simulink library "ddm"  (R2021b)
settings: Solver=VariableStepAuto  StartTime=0.0  StopTime=10.0  RelTol=1e-3
undefined symbols (not defined in the file): ADDM_FrTMTqDev_X_Nm, ADDM_RrTMTqDev_X_Nm, ENUM_ADASACCSTA_ERROR, ENUM_ADASACCSTA_OFF, ENUM_ADASACCSTA_STANDBY, ENUM_ALLOWMOV_ALLOWREADY, ENUM_APS, ENUM_BRKSTA_ERROR, ENUM_BRKSTA_OFF, ENUM_BRKSTA_ON, ENUM_BRKSW_INVALID, ENUM_BRKSW_OFF, ENUM_BRKSW_ON, ENUM_CHGPREACTERRSTA_OBCPRE, ENUM_DCDCFAULTSTA_ANYFAULTLV1, ENUM_DCDCFAULTSTA_ANYFAULTLV2, ENUM_DRIVETRAIN_AWD, ENUM_DRIVETRAIN_FWD, ENUM_DRIVETRAIN_RWD, ENUM_EDUDRTSTA_NORMAL, ENUM_EPBERROR_FAILED, ENUM_EPBSTA_APPLIED, ENUM_EPBSTA_RELEASED, ENUM_ESCAPSSta_APSUNAVAILABLE, ENUM_GEARACTUALPOSN_INVALID, ENUM_GEARACTUALPOSN_P, ENUM_HVBATTREADYPRE_READY, ENUM_HWRESETSTA_HWRESETING, ENUM_MCUWARN_LV0, ENUM_MCUWARN_LV1, ENUM_MCUWARN_LV2, ENUM_MCUWARN_LV3, ENUM_MCUWARN_NOERROR, ENUM_OBCFAULTSTA_ANYFAULT, ENUM_PAS_R2F2, ENUM_PDFAULT_BATTPDFAIL, ENUM_PDFAULT_DCDCDISABLE, ENUM_PDFAULT_MCUDISABLE, ENUM_PDFAULT_MCUDISCHRG, ENUM_POWERSTA_OFF, ENUM_POWERSTA_ON, ENUM_POWERSTA_READY, ENUM_POWERSTA_STANDBY, ENUM_PRESSINDI_LOW, ENUM_PUFAULT_BATTUPFAIL, ENUM_PUFAULT_DCDCENABLEFAIL, ENUM_PUFAULT_PRECHRGCHKFAIL, ENUM_PUFAULT_SAFETYCHKFAIL, ENUM_PWRSTASW_OFF, ENUM_PWRSTASW_OFFA, ENUM_PWRSTASW_OFFCHVCHRG, ENUM_PWRSTASW_OFFCLVCHRG, ENUM_PWRSTASW_ON, ENUM_PWRSTASW_ONHVCHRG, ENUM_PWRSTASW_READY, ENUM_PWRSTASW_STANDBY, ENUM_RAPSErrWarnSta_NORMAL, ENUM_RAPSErrWarnSta_RAPSERRLV1, ENUM_SHIFTCOMMAND_P, ENUM_SHIFTERERRSTA_PBUTTONFAILURE ... (+471)
libraries: hcu_lib x540, simulink x3
(part 14 of 26)

== system ddm/DDM/DDM/TQD/ESC5_DDM ==
  note: Release Condition After Decision
  note: Diagnostics and Fault Handling
  note: Diagnostics and Fault Handling
  note: Release Condition After Decision
  note: Diagnostics and Fault Handling
  note: Release Condition After Decision
  note: ESC5 CheckSum Error (ESC5CSErr)
  note: ESC5 Rolling Count Error (ESC5RCErr)
  note: ESC5 Lost Comm (ESC5NoCom)
  task_time_s : Inport
  VPMM_SysPwrSta_enum : Inport  Port=2
  No_CAN1_BUS_OFF : Inport  Port=3
  VDDM_ESC5NoCom_flg : Inport  Port=4
  VDDM_ESC5RCErr_flg : Inport  Port=5
  VDDM_ESC5CSErr_flg : Inport  Port=6
  DTC_clear_request : Inport  Port=7
  Constant{1,3..5,11,15,18,22,48} (9 alike) : Constant  Value=ENUM_PWRSTASW_OFF
  Constant10 : Constant  Value=ENUM_PWRSTASW_STANDBY
  Constant101 : Constant  Value=KDDM_TQDDiagnosisOffSW_flg
  Constant102 : Constant  Value=ZERO_INT
  Constant12 : Constant  Value=FALSE
  Constant13 : Constant  Value=KDDM_ESC5RCErrDTC_cnt
  Constant14 : Constant  Value=KDDM_ESC5RCErrPassTO_s
  Constant17 : Constant  Value=KDDM_ESC5CSErrDTC_cnt
  Constant2 : Constant  Value=KDDM_ESC5NoComDTC_cnt
  Constant20 : Constant  Value=KDDM_TQDDiagnosisOffSW_flg
  Constant21 : Constant  Value=ENUM_PWRSTASW_STANDBY
  Constant25 : Constant  Value=KDDM_ESC5RCErrDetTO_s
  Constant27 : Constant  Value=FALSE
  Constant28 : Constant  Value=KDDM_ESC5NoComDTC_cnt
  Constant29 : Constant  Value=KDDM_ESC5NoComPassTO_s
  Constant30 : Constant  Value=KDDM_ESC5NoComDetTO_s
  Constant35 : Constant  Value=KDDM_ESC5RCErrPassTO_s
  Constant41 : Constant  Value=FALSE
  Constant42 : Constant  Value=KDDM_ESC5CSErrDTC_cnt
  Constant43 : Constant  Value=KDDM_ESC5CSErrPassTO_s
  Constant44 : Constant  Value=KDDM_ESC5CSErrDetTO_s
  Constant45 : Constant  Value=ZERO_INT
  Constant51 : Constant  Value=KDDM_ESC5CSErrPassTO_s
  Constant55 : Constant  Value=KDDM_ESC5NoComPassTO_s
  Constant6 : Constant  Value=KDDM_ESC5RCErrDTC_cnt
  Constant7 : Constant  Value=KDDM_TQDDiagnosisOffSW_flg
  Constant8 : Constant  Value=ZERO_INT
  Constant9 : Constant  Value=ENUM_PWRSTASW_STANDBY
  DTC_Couter1 : hcu_lib/Basic_Blocks/DTC_Couter
  DTC_Couter2 : hcu_lib/Basic_Blocks/DTC_Couter
  DTC_Couter7 : hcu_lib/Basic_Blocks/DTC_Couter
  DTC_Info1 : hcu_lib/Basic_Blocks/DTC_Info
  DTC_Info2 : hcu_lib/Basic_Blocks/DTC_Info
  DTC_Info3 : hcu_lib/Basic_Blocks/DTC_Info
  Delay1 : Delay  DelayLength=1
  Delay2 : Delay  DelayLength=1
  Delay3 : Delay  DelayLength=1
  Equal{1,7,19,23,49..50} (6 alike) : RelationalOperator  Operator===  OutDataTypeStr=boolean  RndMeth=Simplest
  Equal15 : RelationalOperator  OutDataTypeStr=boolean  RndMeth=Simplest
  Equal{2..6,8} (6 alike) : RelationalOperator  Operator=~=  OutDataTypeStr=boolean  RndMeth=Simplest
  Equal20 : RelationalOperator  OutDataTypeStr=boolean  RndMeth=Simplest
  Equal21 : RelationalOperator  OutDataTypeStr=boolean  RndMeth=Simplest
  Logical Operator : Logic  Operator=OR  Inputs=3  AllPortsSameDT=off  OutDataTypeStr=boolean
  Logical Operator1 : Logic  Operator=OR  Inputs=4  AllPortsSameDT=off  OutDataTypeStr=boolean
  Logical Operator{11..13,19,26,30,37,41,45,53} (10 alike) : Logic  Operator=NOT  AllPortsSameDT=off  OutDataTypeStr=boolean
  Logical Operator{2,5..6,8,54..55} (6 alike) : Logic  AllPortsSameDT=off  OutDataTypeStr=boolean
  Logical Operator{28,32,43,46} (4 alike) : Logic  Inputs=4  AllPortsSameDT=off  OutDataTypeStr=boolean
  Logical Operator3 : Logic  Operator=OR  Inputs=4  AllPortsSameDT=off  OutDataTypeStr=boolean
  Logical Operator4 : Logic  Inputs=3  AllPortsSameDT=off  OutDataTypeStr=boolean
  Logical Operator49 : Logic  Operator=OR  Inputs=4  AllPortsSameDT=off  OutDataTypeStr=boolean
  Logical Operator50 : Logic  Inputs=3  AllPortsSameDT=off  OutDataTypeStr=boolean
  NOT1 : Logic  Operator=NOT  AllPortsSameDT=off  OutDataTypeStr=boolean
  NOT2 : Logic  Operator=NOT  AllPortsSameDT=off  OutDataTypeStr=boolean
  NOT3 : Logic  Operator=NOT  AllPortsSameDT=off  OutDataTypeStr=boolean
  Relational Operator1 : RelationalOperator  Operator=>  OutDataTypeStr=boolean  RndMeth=Simplest
  Relational Operator2 : RelationalOperator  Operator=>  OutDataTypeStr=boolean  RndMeth=Simplest
  Relational Operator3 : RelationalOperator  Operator=>  OutDataTypeStr=boolean  RndMeth=Simplest
  Switch1 : Switch  Criteria=u2 ~= 0
  Switch2 : Switch  Criteria=u2 ~= 0
  Switch3 : Switch  Criteria=u2 ~= 0
  Terminator : Terminator
  Terminator1 : Terminator
  Terminator2 : Terminator
  Test Detection Criteria2 : hcu_lib/Basic_Blocks/Test Detection Criteria
  Test Detection Criteria3 : hcu_lib/Basic_Blocks/Test Detection Criteria
  Test Detection Criteria4 : hcu_lib/Basic_Blocks/Test Detection Criteria
  Timer1 : hcu_lib/Basic_Blocks/Timer
  Timer3 : hcu_lib/Basic_Blocks/Timer
  Timer4 : hcu_lib/Basic_Blocks/Timer
  Unit Delay1 : UnitDelay  SampleTime=-1  HasFrameUpgradeWarning=on
  Unit Delay6 : UnitDelay  SampleTime=-1  HasFrameUpgradeWarning=on
  Unit Delay7 : UnitDelay  SampleTime=-1  HasFrameUpgradeWarning=on
  VDDM_ESC5NoComDTC_raw32 : Outport
  VDDM_ESC5RCErrDTC_raw32 : Outport  Port=2
  VDDM_ESC5CSErrDTC_raw32 : Outport  Port=3
  VDDM_ESC5NoComCFS_flg : Outport  Port=4
  VDDM_ESC5RCErrCFS_flg : Outport  Port=5
  VDDM_ESC5CSErrCFS_flg : Outport  Port=6
  VDDM_ESC5Err_flg : Outport  Port=7
  wires:
  [VPMM_SysPwrSta_enum] -> Equal8/1
  Constant15/1 -> Equal8/2
  [VPMM_SysPwrSta_enum] -> Equal5/1
  Constant11/1 -> Equal5/2
  Equal7/1 -> Logical Operator2/1
  [VDDM_ESC5CSErrCFS_flg] -> Delay2/1
  Constant18/1 -> Equal7/2
  DTC_Couter2/2 -> Relational Operator1/1  "VDDM_ESC5CSErrDTC_cnt"
  [VDDM_ESC5CSErrCFSRls_flg] -> DTC_Couter2/2
  [DTC_clear_request] -> Logical Operator1/2
  Equal1/1 -> Logical Operator2/2
  Delay2/1 -> NOT2/1
  Logical Operator6/1 -> Logical Operator1/3
  Constant8/1 -> Relational Operator1/2
  Constant7/1 -> Logical Operator1/4
  Unit Delay1/1 -> Equal7/1
  Relational Operator1/1 -> Terminator2/1  "VDDM_ESC5CSErrDFS_flg"
  [VDDM_ESC5CSErrPass_flg] -> Logical Operator6/1
  DTC_Couter2/1 -> [VDDM_ESC5CSErrCFS_flg]  "VDDM_ESC5CSErrCFS_flg"
  [VPMM_SysPwrSta_enum] -> Unit Delay1/1
  Logical Operator2/1 -> Logical Operator1/1
  Constant10/1 -> Equal1/2
  NOT2/1 -> Logical Operator6/2
  [VPMM_SysPwrSta_enum] -> Equal1/1
  Constant17/1 -> DTC_Couter2/3
  Logical Operator1/1 -> [VDDM_ESC5CSErrCFSRls_flg]  "VDDM_ESC5CSErrCFSRls_flg"
  [VDDM_ESC5CSErrDet_flg] -> DTC_Couter2/1
  Equal49/1 -> Logical Operator5/2
  [VPMM_SysPwrSta_enum] -> Equal49/1
  NOT3/1 -> Logical Operator8/2
  DTC_Couter7/1 -> [VDDM_ESC5RCErrCFS_flg]  "VDDM_ESC5RCErrCFS_flg"
  Constant9/1 -> Equal49/2
  [VPMM_SysPwrSta_enum] -> Unit Delay7/1
  Equal50/1 -> Logical Operator5/1
  Relational Operator3/1 -> Terminator1/1  "VDDM_ESC5RCErrDFS_flg"
  [VDDM_ESC5RCErrPass_flg] -> Logical Operator8/1
  Logical Operator5/1 -> Logical Operator3/1
  [VDDM_ESC5RCErrCFS_flg] -> Delay3/1
  Logical Operator8/1 -> Logical Operator3/3
  Constant101/1 -> Logical Operator3/4
  [DTC_clear_request] -> Logical Operator3/2
  Constant102/1 -> Relational Operator3/2
  Constant6/1 -> DTC_Couter7/3
  [VDDM_ESC5RCErrDet_flg] -> DTC_Couter7/1
  Logical Operator3/1 -> [VDDM_ESC5RCErrCFSRls_flg]  "VDDM_ESC5RCErrCFSRls_flg"
  DTC_Couter7/2 -> Relational Operator3/1  "VDDM_ESC5RCErrDTC_cnt"
  Delay3/1 -> NOT3/1
  [VDDM_ESC5RCErrCFSRls_flg] -> DTC_Couter7/2
  Constant22/1 -> Equal50/2
  Unit Delay7/1 -> Equal50/1
  Constant5/1 -> Equal6/2
  [VPMM_SysPwrSta_enum] -> Equal6/1
  Constant4/1 -> Equal4/2
  [VPMM_SysPwrSta_enum] -> Equal4/1
  [VPMM_SysPwrSta_enum] -> Equal3/1
  Constant1/1 -> Equal3/2
  [VPMM_SysPwrSta_enum] -> Equal2/1
  Constant3/1 -> Equal2/2
  Equal19/1 -> Logical Operator55/2
  [VDDM_ESC5NoComPass_flg] -> Logical Operator54/1
  Constant2/1 -> DTC_Couter1/3
  [VDDM_ESC5NoComCFS_flg] -> Delay1/1
  DTC_Couter1/2 -> Relational Operator2/1  "VDDM_ESC5NoComDTC_cnt"
  DTC_Couter1/1 -> [VDDM_ESC5NoComCFS_flg]  "VDDM_ESC5NoComCFS_flg"
  Constant21/1 -> Equal19/2
  Equal23/1 -> Logical Operator55/1
  [VPMM_SysPwrSta_enum] -> Equal19/1
  [VDDM_ESC5NoComCFSRls_flg] -> DTC_Couter1/2
  [VDDM_ESC5NoComDet_flg] -> DTC_Couter1/1
  Constant48/1 -> Equal23/2
  Unit Delay6/1 -> Equal23/1
  Logical Operator49/1 -> [VDDM_ESC5NoComCFSRls_flg]  "VDDM_ESC5NoComCFSRls_flg"
  [DTC_clear_request] -> Logical Operator49/2
  Constant45/1 -> Relational Operator2/2
  Relational Operator2/1 -> Terminator/1  "VDDM_ESC5NoComDFS_flg"
  Logical Operator54/1 -> Logical Operator49/3
  Delay1/1 -> NOT1/1
  NOT1/1 -> Logical Operator54/2
  Constant20/1 -> Logical Operator49/4
  Logical Operator55/1 -> Logical Operator49/1
  [VPMM_SysPwrSta_enum] -> Unit Delay6/1
  [VDDM_ESC5CSErrCFS_flg] -> VDDM_ESC5CSErrCFS_flg/1
  [VDDM_ESC5RCErrCFS_flg] -> VDDM_ESC5RCErrCFS_flg/1
  [VDDM_ESC5NoComCFS_flg] -> VDDM_ESC5NoComCFS_flg/1
  [VDDM_ESC5NoComCFS_flg] -> Logical Operator13/1
  Logical Operator13/1 -> Logical Operator43/4
  [VDDM_ESC5NoComCFS_flg] -> Logical Operator11/1
  Logical Operator11/1 -> Logical Operator28/4
  VDDM_ESC5CSErr_flg/1 -> [VDDM_ESC5CSErr_flg]
  VDDM_ESC5RCErr_flg/1 -> [VDDM_ESC5RCErr_flg]
  [VDDM_ESC5NoCom_flg] -> Logical Operator4/3
  Test Detection Criteria2/1 -> [VDDM_ESC5NoComDet_flg]  "VDDM_ESC5NoComDet_flg"
  Logical Operator37/1 -> Timer4/2
  Test Detection Criteria3/1 -> [VDDM_ESC5RCErrDet_flg]  "VDDM_ESC5RCErrDet_flg"
  [No_CAN1_BUS_OFF] -> Logical Operator32/2
  [No_CAN1_BUS_OFF] -> Logical Operator50/2
  [VDDM_ESC5NoCom_flg] -> Logical Operator53/1
  [VDDM_ESC5NoComPass_flg] -> DTC_Info1/2
  VDDM_ESC5NoCom_flg/1 -> [VDDM_ESC5NoCom_flg]
  Switch3/1 -> Test Detection Criteria2/1
  Timer4/1 -> Equal15/1
  Logical Operator41/1 -> Logical Operator32/4
  [VDDM_ESC5RCErr_flg] -> Logical Operator30/1
  Logical Operator19/1 -> Timer3/2
  Equal21/1 -> [VDDM_ESC5RCErrPass_flg]  "VDDM_ESC5RCErrPass_flg"
  Logical Operator43/1 -> Logical Operator37/1, Timer4/1
  Logical Operator53/1 -> Logical Operator50/3
  Logical Operator46/1 -> Switch1/3
  Constant44/1 -> Test Detection Criteria4/4
  [VDDM_ESC5CSErrCFS_flg] -> DTC_Info3/3
  Logical Operator26/1 -> Logical Operator46/4
  [VDDM_ESC5RCErrCFSRls_flg] -> Switch1/2
  [task_time_s] -> Timer4/3
  Constant12/1 -> Switch1/1
  Logical Operator12/1 -> Timer1/2
  [No_CAN1_BUS_OFF] -> Logical Operator4/2
  Logical Operator4/1 -> Switch3/3
  [task_time_s] -> Test Detection Criteria3/2
  [VDDM_ESC5RCErrDet_flg] -> DTC_Info2/1
  [task_time_s] -> Test Detection Criteria4/2
  Logical Operator28/1 -> Logical Operator12/1, Timer1/1
  Equal2/1 -> Logical Operator4/1
  DTC_Info1/1 -> VDDM_ESC5NoComDTC_raw32/1  "VDDM_ESC5NoComDTC_raw32"
  Constant13/1 -> Test Detection Criteria3/3
  Test Detection Criteria4/1 -> [VDDM_ESC5CSErrDet_flg]  "VDDM_ESC5CSErrDet_flg"
  Switch1/1 -> Test Detection Criteria3/1
  [VDDM_ESC5RCErr_flg] -> Logical Operator46/3
  Equal5/1 -> Logical Operator32/1
  [VDDM_ESC5CSErrDet_flg] -> DTC_Info3/1
  Logical Operator50/1 -> Timer3/1, Logical Operator19/1
  No_CAN1_BUS_OFF/1 -> [No_CAN1_BUS_OFF]
  [VDDM_ESC5NoComCFS_flg] -> Logical Operator26/1
  [DTC_clear_request] -> DTC_Info3/4
  Equal3/1 -> Logical Operator50/1
  [VDDM_ESC5CSErrCFSRls_flg] -> Switch2/2
  Constant42/1 -> Test Detection Criteria4/3
  [VDDM_ESC5NoComCFS_flg] -> Logical Operator41/1
  DTC_clear_request/1 -> [DTC_clear_request]
  [VDDM_ESC5RCErrCFS_flg] -> DTC_Info2/3
  Constant35/1 -> Timer1/4
  Logical Operator30/1 -> Logical Operator28/3
  Timer1/1 -> Equal21/1
  [VDDM_ESC5NoComDet_flg] -> DTC_Info1/1
  Equal6/1 -> Logical Operator28/1
  [No_CAN1_BUS_OFF] -> Logical Operator28/2
  Constant14/1 -> Equal21/2
  Logical Operator32/1 -> Switch2/3
  Equal20/1 -> [VDDM_ESC5NoComPass_flg]  "VDDM_ESC5NoComPass_flg"
  [VDDM_ESC5RCErrPass_flg] -> DTC_Info2/2
  [task_time_s] -> Timer1/3
  [VDDM_ESC5NoComCFSRls_flg] -> Switch3/2
  VPMM_SysPwrSta_enum/1 -> [VPMM_SysPwrSta_enum]
  Equal4/1 -> Logical Operator46/1
  Constant51/1 -> Timer4/4
  Switch2/1 -> Test Detection Criteria4/1
  [VDDM_ESC5CSErrPass_flg] -> DTC_Info3/2
  Equal15/1 -> [VDDM_ESC5CSErrPass_flg]  "VDDM_ESC5CSErrPass_flg"
  Constant43/1 -> Equal15/2
  Constant30/1 -> Test Detection Criteria2/4
  Constant28/1 -> Test Detection Criteria2/3
  [DTC_clear_request] -> DTC_Info2/4
  Constant25/1 -> Test Detection Criteria3/4
  [task_time_s] -> Timer3/3
  DTC_Info3/1 -> VDDM_ESC5CSErrDTC_raw32/1  "VDDM_ESC5CSErrDTC_raw32"
  [task_time_s] -> Test Detection Criteria2/2
  [VDDM_ESC5NoComCFS_flg] -> DTC_Info1/3
  [No_CAN1_BUS_OFF] -> Logical Operator43/2
  [VDDM_ESC5CSErr_flg] -> Logical Operator45/1
  DTC_Info2/1 -> VDDM_ESC5RCErrDTC_raw32/1  "VDDM_ESC5RCErrDTC_raw32"
  Equal8/1 -> Logical Operator43/1
  task_time_s/1 -> [task_time_s]
  Constant27/1 -> Switch3/1
  Constant29/1 -> Equal20/2
  Logical Operator45/1 -> Logical Operator43/3
  Constant41/1 -> Switch2/1
  [No_CAN1_BUS_OFF] -> Logical Operator46/2
  [DTC_clear_request] -> DTC_Info1/4
  Timer3/1 -> Equal20/1
  Constant55/1 -> Timer3/4
  [VDDM_ESC5CSErr_flg] -> Logical Operator32/3
  [VDDM_ESC5RCErrCFS_flg] -> Logical Operator/2
  [VDDM_ESC5NoComCFS_flg] -> Logical Operator/1
  [VDDM_ESC5CSErrCFS_flg] -> Logical Operator/3
  Logical Operator/1 -> VDDM_ESC5Err_flg/1  "VDDM_ESC5Err_flg"

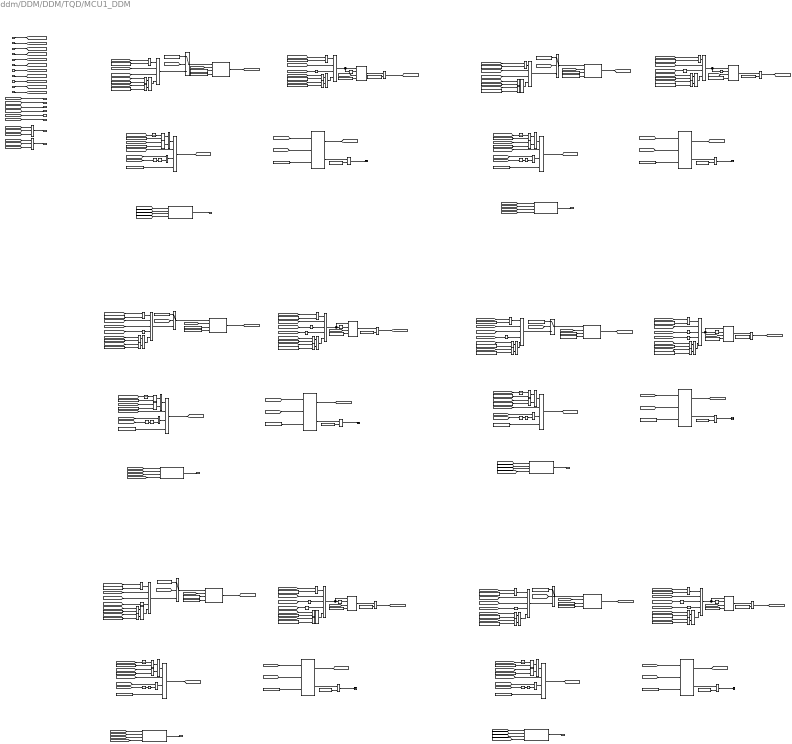
== system ddm/DDM/DDM/TQD/MCU1_DDM ==
  note: Diagnostics and Fault Handling
  note: Release Condition After Decision
  note: Diagnostics and Fault Handling
  note: Release Condition After Decision
  note: Diagnostics and Fault Handling
  note: Release Condition After Decision
  note: Release Condition After Decision
  note: Diagnostics and Fault Handling
  note: Release Condition After Decision
  note: Diagnostics and Fault Handling
  note: Release Condition After Decision
  note: Diagnostics and Fault Handling
  note: MCU_F1 Lost Comm (MCUF1NoCom)
  note: MCU_R1 Lost Comm (MCUR1NoCom)
  note: MCU_R1 Rolling Count Error (MCUR1RCErr)
  note: MCU_F1 Rolling Count Error (MCUF1RCErr)
  note: MCU_R1 Checksum Error (MCUR1CSErr)
  note: MCU_F1 Checksum Error (MCUF1CSErr)
  task_time_s : Inport
  VPMM_SysPwrSta_enum : Inport  Port=2
  No_CAN3_BUS_OFF : Inport  Port=3
  VDDM_MCUF1NoCom_flg : Inport  Port=4
  VDDM_MCUR1NoCom_flg : Inport  Port=5
  VDDM_MCUF1RCErr_flg : Inport  Port=6
  VDDM_MCUF1CSErr_flg : Inport  Port=7
  VDDM_MCUR1RCErr_flg : Inport  Port=8
  VDDM_MCUR1CSErr_flg : Inport  Port=9
  DTC_clear_request : Inport  Port=10
  VPMM_DrivetrainSelect_enum : Inport  Port=11
  Constant{1..2,6..7,9,13,26,40,43,46,53,59..60,62,72,75,79,86} (18 alike) : Constant  Value=ENUM_PWRSTASW_OFF
  Constant{3,10,35,41,52,57} (6 alike) : Constant  Value=ENUM_PWRSTASW_STANDBY
  Constant{20,24,28,44,67,88,90,92,94,96,98,100} (12 alike) : Constant  Value=ENUM_DRIVETRAIN_AWD
  Constant{4,11,29,45,55,101} (6 alike) : Constant  Value=KDDM_TQDDiagnosisOffSW_flg
  Constant{5,12,30,49,56,102} (6 alike) : Constant  Value=ZERO_INT
  Constant14 : Constant  Value=KDDM_MCUF1NoComDTC_cnt
  Constant{15,27,66,93,95,97} (6 alike) : Constant  Value=ENUM_DRIVETRAIN_RWD
  Constant16 : Constant  Value=KDDM_MCUR1NoComDTC_cnt
  Constant17 : Constant  Value=KDDM_MCUR1NoComPassTO_s
  Constant18 : Constant  Value=KDDM_MCUR1NoComPassTO_s
  Constant19 : Constant  Value=KDDM_MCUR1NoComDetTO_s
  Constant{21,42,87,89,91,99} (6 alike) : Constant  Value=ENUM_DRIVETRAIN_FWD
  Constant{22..23,38..39,73..74} (6 alike) : Constant  Value=FALSE
  Constant25 : Constant  Value=KDDM_MCUF1RCErrDTC_cnt
  Constant31 : Constant  Value=KDDM_MCUR1RCErrDTC_cnt
  Constant32 : Constant  Value=KDDM_MCUR1RCErrPassTO_s
  Constant33 : Constant  Value=KDDM_MCUR1RCErrPassTO_s
  Constant34 : Constant  Value=KDDM_MCUR1RCErrDetTO_s
  Constant36 : Constant  Value=KDDM_MCUR1RCErrDTC_cnt
  Constant37 : Constant  Value=KDDM_MCUF1CSErrPassTO_s
  Constant47 : Constant  Value=KDDM_MCUF1RCErrDTC_cnt
  Constant48 : Constant  Value=KDDM_MCUF1RCErrPassTO_s
  Constant50 : Constant  Value=KDDM_MCUF1RCErrPassTO_s
  Constant51 : Constant  Value=KDDM_MCUF1RCErrDetTO_s
  Constant54 : Constant  Value=KDDM_MCUF1RCErrDTC_cnt
  Constant58 : Constant  Value=KDDM_MCUR1RCErrDTC_cnt
  Constant61 : Constant  Value=KDDM_MCUR1CSErrDTC_cnt
  Constant63 : Constant  Value=KDDM_MCUR1CSErrPassTO_s
  Constant64 : Constant  Value=KDDM_MCUR1CSErrPassTO_s
  Constant65 : Constant  Value=KDDM_MCUR1CSErrDetTO_s
  Constant68 : Constant  Value=KDDM_MCUF1NoComDTC_cnt
  Constant69 : Constant  Value=KDDM_MCUF1NoComPassTO_s
  Constant70 : Constant  Value=KDDM_MCUF1NoComPassTO_s
  Constant71 : Constant  Value=KDDM_MCUF1NoComDetTO_s
  Constant8 : Constant  Value=KDDM_MCUR1NoComDTC_cnt
  Constant80 : Constant  Value=KDDM_MCUF1CSErrDTC_cnt
  Constant83 : Constant  Value=KDDM_MCUF1CSErrPassTO_s
  Constant84 : Constant  Value=KDDM_MCUF1CSErrDetTO_s
  DTC_Couter{1..5,7} (6 alike) : hcu_lib/Basic_Blocks/DTC_Couter
  DTC_Info{,1..5} (6 alike) : hcu_lib/Basic_Blocks/DTC_Info
  Delay{1..6} (6 alike) : Delay  DelayLength=1
  Equal{,1..4,7..8,12,14..15,19..20,23,26..27,33..43,45,47..55} (36 alike) : RelationalOperator  Operator===  OutDataTypeStr=boolean  RndMeth=Simplest
  Equal{5,9..11,16,18,21..22,24,29,44,46} (12 alike) : RelationalOperator  Operator=~=  OutDataTypeStr=boolean  RndMeth=Simplest
  Equal{6,13,17,25,28,30} (6 alike) : RelationalOperator  OutDataTypeStr=boolean  RndMeth=Simplest
  Logical Operator : Logic  Operator=OR  Inputs=3  AllPortsSameDT=off  OutDataTypeStr=boolean
  Logical Operator{1,3,16,21,33,36} (6 alike) : Logic  Operator=OR  Inputs=4  AllPortsSameDT=off  OutDataTypeStr=boolean
  Logical Operator{6,10,13,15,19..20,24..26,29,32,37,41..42,61,70,81..84} (20 alike) : Logic  Operator=NOT  AllPortsSameDT=off  OutDataTypeStr=boolean
  Logical Operator{4,8..9,11,17..18,22,28,34..35,38..39} (12 alike) : Logic  AllPortsSameDT=off  OutDataTypeStr=boolean
  Logical Operator{7,12,23,27,31,40,58,67} (8 alike) : Logic  Inputs=5  AllPortsSameDT=off  OutDataTypeStr=boolean
  Logical Operator{2,5,14,30} (4 alike) : Logic  Inputs=4  AllPortsSameDT=off  OutDataTypeStr=boolean
  Logical Operator43 : Logic  Operator=OR  Inputs=3  AllPortsSameDT=off  OutDataTypeStr=boolean
  NOT{1..6} (6 alike) : Logic  Operator=NOT  AllPortsSameDT=off  OutDataTypeStr=boolean
  OR{,1..11} (12 alike) : Logic  Operator=OR  AllPortsSameDT=off  OutDataTypeStr=boolean
  Relational Operator{1..6} (6 alike) : RelationalOperator  Operator=>  OutDataTypeStr=boolean  RndMeth=Simplest
  Switch{1..6} (6 alike) : Switch  Criteria=u2 ~= 0
  Terminator{,1..5} (6 alike) : Terminator
  Test Detection Criteria{1..6} (6 alike) : hcu_lib/Basic_Blocks/Test Detection Criteria
  Timer{1..6} (6 alike) : hcu_lib/Basic_Blocks/Timer
  Unit Delay{1..4,6..7} (6 alike) : UnitDelay  SampleTime=-1  HasFrameUpgradeWarning=on
  VDDM_MCUF1NoComDTC_raw32 : Outport
  VDDM_MCUR1NoComDTC_raw32 : Outport  Port=2
  VDDM_MCUF1RCErrDTC_raw32 : Outport  Port=3
  VDDM_MCUR1RCErrDTC_raw32 : Outport  Port=4
  VDDM_MCUF1CSErrDTC_raw32 : Outport  Port=5
  VDDM_MCUR1CSErrDTC_raw32 : Outport  Port=6
  VDDM_MCUF1NoComCFS_flg : Outport  Port=7
  VDDM_MCUF1RCErrCFS_flg : Outport  Port=8
  VDDM_MCUF1CSErrCFS_flg : Outport  Port=9
  VDDM_MCUR1NoComCFS_flg : Outport  Port=10
  VDDM_MCUR1RCErrCFS_flg : Outport  Port=11
  VDDM_MCUR1CSErrCFS_flg : Outport  Port=12
  VDDM_MCUF1Err_flg : Outport  Port=13
  VDDM_MCUR1Err_flg : Outport  Port=14
  wires:
  Logical Operator42/1 -> Logical Operator40/3
  [VDDM_MCUR1CSErr_flg] -> Logical Operator42/1
  [VPMM_DrivetrainSelect_enum] -> Equal54/1
  Logical Operator41/1 -> Logical Operator40/4
  Constant67/1 -> Equal55/2
  [VPMM_DrivetrainSelect_enum] -> Equal55/1
  Equal22/1 -> Logical Operator40/1
  Constant66/1 -> Equal54/2
  OR11/1 -> Logical Operator40/5
  Equal55/1 -> OR11/2
  [No_CAN3_BUS_OFF] -> Logical Operator40/2
  Constant60/1 -> Equal22/2
  [VDDM_MCUR1NoComCFS_flg] -> Logical Operator41/1
  Equal54/1 -> OR11/1
  [VPMM_SysPwrSta_enum] -> Equal22/1
  [VPMM_SysPwrSta_enum] -> Unit Delay4/1
  NOT6/1 -> Logical Operator39/2
  [VDDM_MCUR1CSErrPass_flg] -> Logical Operator39/1
  DTC_Couter5/2 -> Relational Operator6/1  "VDDM_MCUR1CSErrDTC_cnt"
  Constant59/1 -> Equal27/2
  Relational Operator6/1 -> Terminator5/1  "VDDM_MCUR1CSErrDFS_flg"
  Delay6/1 -> NOT6/1
  Unit Delay4/1 -> Equal27/1
  Constant58/1 -> DTC_Couter5/3
  Equal26/1 -> Logical Operator38/2
  Equal27/1 -> Logical Operator38/1
  [VPMM_SysPwrSta_enum] -> Equal26/1
  Logical Operator39/1 -> Logical Operator36/3
  Constant55/1 -> Logical Operator36/4
  Constant57/1 -> Equal26/2
  Logical Operator38/1 -> Logical Operator36/1
  Logical Operator36/1 -> [VDDM_MCUR1CSErrCFSRls_flg]  "VDDM_MCUR1CSErrCFSRls_flg"
  Constant56/1 -> Relational Operator6/2
  [VDDM_MCUR1CSErrDet_flg] -> DTC_Couter5/1
  [DTC_clear_request] -> Logical Operator36/2
  [VDDM_MCUR1CSErrCFS_flg] -> Delay6/1
  DTC_Couter5/1 -> [VDDM_MCUR1CSErrCFS_flg]  "VDDM_MCUR1CSErrCFS_flg"
  [VDDM_MCUR1CSErrCFSRls_flg] -> DTC_Couter5/2
  [VPMM_SysPwrSta_enum] -> Equal52/1
  Constant75/1 -> Equal53/2
  [VDDM_MCUF1CSErrDet_flg] -> DTC_Couter4/1
  Delay5/1 -> NOT5/1
  Unit Delay3/1 -> Equal53/1
  [VDDM_MCUF1CSErrCFSRls_flg] -> DTC_Couter4/2
  Constant54/1 -> DTC_Couter4/3
  Equal53/1 -> Logical Operator34/1
  Equal52/1 -> Logical Operator34/2
  [VPMM_SysPwrSta_enum] -> Unit Delay3/1
  NOT5/1 -> Logical Operator35/2
  Logical Operator34/1 -> Logical Operator33/1
  Constant52/1 -> Equal52/2
  Constant45/1 -> Logical Operator33/4
  [DTC_clear_request] -> Logical Operator33/2
  Logical Operator35/1 -> Logical Operator33/3
  DTC_Couter4/2 -> Relational Operator5/1  "VDDM_MCUF1CSErrDTC_cnt"
  [VDDM_MCUF1CSErrPass_flg] -> Logical Operator35/1
  Logical Operator33/1 -> [VDDM_MCUF1CSErrCFSRls_flg]  "VDDM_MCUF1CSErrCFSRls_flg"
  Constant49/1 -> Relational Operator5/2
  Relational Operator5/1 -> Terminator4/1  "VDDM_MCUF1CSErrDFS_flg"
  DTC_Couter4/1 -> [VDDM_MCUF1CSErrCFS_flg]  "VDDM_MCUF1CSErrCFS_flg"
  [VDDM_MCUF1CSErrCFS_flg] -> Delay5/1
  Logical Operator32/1 -> Logical Operator27/3
  OR10/1 -> Logical Operator27/5
  Equal20/1 -> OR10/2
  Equal19/1 -> OR10/1
  [VPMM_DrivetrainSelect_enum] -> Equal19/1
  Constant42/1 -> Equal19/2
  Constant44/1 -> Equal20/2
  [VPMM_DrivetrainSelect_enum] -> Equal20/1
  [VDDM_MCUF1NoComCFS_flg] -> Logical Operator29/1
  Logical Operator29/1 -> Logical Operator27/4
  [VDDM_MCUF1CSErr_flg] -> Logical Operator32/1
  Constant40/1 -> Equal18/2
  Equal18/1 -> Logical Operator27/1
  [No_CAN3_BUS_OFF] -> Logical Operator27/2
  [VPMM_SysPwrSta_enum] -> Equal18/1
  Logical Operator6/1 -> Logical Operator5/3
  Logical Operator25/1 -> Timer2/2
  Logical Operator24/1 -> Logical Operator2/3
  Logical Operator10/1 -> Timer1/2
  [VPMM_SysPwrSta_enum] -> Equal15/1
  Constant43/1 -> Equal51/2
  [VDDM_MCUR1RCErrDet_flg] -> DTC_Couter3/1
  Delay4/1 -> NOT4/1
  Unit Delay2/1 -> Equal51/1
  [VDDM_MCUR1RCErrCFSRls_flg] -> DTC_Couter3/2
  Constant36/1 -> DTC_Couter3/3
  Equal51/1 -> Logical Operator22/1
  Equal15/1 -> Logical Operator22/2
  [VPMM_SysPwrSta_enum] -> Unit Delay2/1
  NOT4/1 -> Logical Operator28/2
  Logical Operator22/1 -> Logical Operator21/1
  Constant35/1 -> Equal15/2
  Constant29/1 -> Logical Operator21/4
  [DTC_clear_request] -> Logical Operator21/2
  Logical Operator28/1 -> Logical Operator21/3
  DTC_Couter3/2 -> Relational Operator4/1  "VDDM_MCUR1RCErrDTC_cnt"
  [VDDM_MCUR1RCErrPass_flg] -> Logical Operator28/1
  Logical Operator21/1 -> [VDDM_MCUR1RCErrCFSRls_flg]  "VDDM_MCUR1RCErrCFSRls_flg"
  Constant30/1 -> Relational Operator4/2
  Relational Operator4/1 -> Terminator3/1  "VDDM_MCUR1RCErrDFS_flg"
  DTC_Couter3/1 -> [VDDM_MCUR1RCErrCFS_flg]  "VDDM_MCUR1RCErrCFS_flg"
  [VDDM_MCUR1RCErrCFS_flg] -> Delay4/1
  Logical Operator20/1 -> Logical Operator7/3
  OR9/1 -> Logical Operator7/5
  [VPMM_DrivetrainSelect_enum] -> Equal14/1
  Constant27/1 -> Equal12/2
  Equal14/1 -> OR9/2
  [VPMM_DrivetrainSelect_enum] -> Equal12/1
  Constant28/1 -> Equal14/2
  Equal12/1 -> OR9/1
  [VDDM_MCUR1NoComCFS_flg] -> Logical Operator19/1
  Logical Operator19/1 -> Logical Operator7/4
  [No_CAN3_BUS_OFF] -> Logical Operator7/2
  Equal10/1 -> Logical Operator7/1
  Constant26/1 -> Equal10/2
  [VDDM_MCUR1RCErr_flg] -> Logical Operator20/1
  [VPMM_SysPwrSta_enum] -> Equal10/1
  Delay3/1 -> NOT3/1
  [VDDM_MCUF1RCErrCFS_flg] -> Delay3/1
  Constant101/1 -> Logical Operator16/4
  [DTC_clear_request] -> Logical Operator16/2
  NOT3/1 -> Logical Operator18/2
  Constant41/1 -> Equal49/2
  Logical Operator17/1 -> Logical Operator16/1
  [VPMM_SysPwrSta_enum] -> Unit Delay7/1
  Relational Operator3/1 -> Terminator2/1  "VDDM_MCUF1RCErrDFS_flg"
  Equal49/1 -> Logical Operator17/2
  Constant72/1 -> Equal50/2
  Unit Delay7/1 -> Equal50/1
  [VPMM_SysPwrSta_enum] -> Equal49/1
  Equal50/1 -> Logical Operator17/1
  [VDDM_MCUF1RCErrPass_flg] -> Logical Operator18/1
  Logical Operator18/1 -> Logical Operator16/3
  Constant25/1 -> DTC_Couter7/3
  DTC_Couter7/1 -> [VDDM_MCUF1RCErrCFS_flg]  "VDDM_MCUF1RCErrCFS_flg"
  Logical Operator16/1 -> [VDDM_MCUF1RCErrCFSRls_flg]  "VDDM_MCUF1RCErrCFSRls_flg"
  [VDDM_MCUF1RCErrCFSRls_flg] -> DTC_Couter7/2
  DTC_Couter7/2 -> Relational Operator3/1  "VDDM_MCUF1RCErrDTC_cnt"
  [VDDM_MCUF1RCErrDet_flg] -> DTC_Couter7/1
  Constant102/1 -> Relational Operator3/2
  Logical Operator15/1 -> Logical Operator12/3
  [VPMM_DrivetrainSelect_enum] -> Equal48/1
  Constant24/1 -> Equal48/2
  [VDDM_MCUF1NoComCFS_flg] -> Logical Operator13/1
  Equal47/1 -> OR8/1
  [VPMM_SysPwrSta_enum] -> Equal9/1
  Logical Operator13/1 -> Logical Operator12/4
  Constant21/1 -> Equal47/2
  Equal9/1 -> Logical Operator12/1
  Equal48/1 -> OR8/2
  [VPMM_DrivetrainSelect_enum] -> Equal47/1
  OR8/1 -> Logical Operator12/5
  [VDDM_MCUF1RCErr_flg] -> Logical Operator15/1
  Constant7/1 -> Equal9/2
  [No_CAN3_BUS_OFF] -> Logical Operator12/2
  Delay2/1 -> NOT2/1
  [VDDM_MCUR1NoComCFS_flg] -> Delay2/1
  Constant4/1 -> Logical Operator1/4
  [DTC_clear_request] -> Logical Operator1/2
  NOT2/1 -> Logical Operator11/2
  Constant3/1 -> Equal7/2
  Logical Operator9/1 -> Logical Operator1/1
  [VPMM_SysPwrSta_enum] -> Unit Delay1/1
  Relational Operator1/1 -> Terminator1/1  "VDDM_MCUR1NoComDFS_flg"
  Equal7/1 -> Logical Operator9/2
  Constant6/1 -> Equal8/2
  Unit Delay1/1 -> Equal8/1
  [VPMM_SysPwrSta_enum] -> Equal7/1
  Equal8/1 -> Logical Operator9/1
  [VDDM_MCUR1NoComPass_flg] -> Logical Operator11/1
  Logical Operator11/1 -> Logical Operator1/3
  Constant8/1 -> DTC_Couter2/3
  DTC_Couter2/1 -> [VDDM_MCUR1NoComCFS_flg]  "VDDM_MCUR1NoComCFS_flg"
  Logical Operator1/1 -> [VDDM_MCUR1NoComCFSRls_flg]  "VDDM_MCUR1NoComCFSRls_flg"
  [VDDM_MCUR1NoComCFSRls_flg] -> DTC_Couter2/2
  DTC_Couter2/2 -> Relational Operator1/1  "VDDM_MCUR1NoComDTC_cnt"
  [VDDM_MCUR1NoComDet_flg] -> DTC_Couter2/1
  Constant5/1 -> Relational Operator1/2
  Logical Operator5/1 -> Logical Operator25/1, Timer2/1
  Equal2/1 -> OR7/1
  Constant20/1 -> Equal23/2
  OR7/1 -> Logical Operator5/4
  [VPMM_DrivetrainSelect_enum] -> Equal2/1
  Equal23/1 -> OR7/2
  Constant15/1 -> Equal2/2
  [VPMM_DrivetrainSelect_enum] -> Equal23/1
  [No_CAN3_BUS_OFF] -> Logical Operator5/2
  Constant2/1 -> Equal46/2
  [VDDM_MCUR1NoCom_flg] -> Logical Operator6/1
  Equal46/1 -> Logical Operator5/1
  [VPMM_SysPwrSta_enum] -> Equal46/1
  Constant13/1 -> Equal4/2
  [VPMM_SysPwrSta_enum] -> Equal3/1
  Constant10/1 -> Equal3/2
  Equal4/1 -> Logical Operator4/1
  [DTC_clear_request] -> Logical Operator3/2
  Logical Operator8/1 -> Logical Operator3/3
  Logical Operator4/1 -> Logical Operator3/1
  [VDDM_MCUF1NoComPass_flg] -> Logical Operator8/1
  Constant11/1 -> Logical Operator3/4
  Logical Operator3/1 -> [VDDM_MCUF1NoComCFSRls_flg]  "VDDM_MCUF1NoComCFSRls_flg"
  NOT1/1 -> Logical Operator8/2
  [VDDM_MCUF1NoComCFS_flg] -> Delay1/1
  Delay1/1 -> NOT1/1
  Equal3/1 -> Logical Operator4/2
  Unit Delay6/1 -> Equal4/1
  [VPMM_SysPwrSta_enum] -> Unit Delay6/1
  DTC_Couter1/2 -> Relational Operator2/1  "VDDM_MCUF1NoComDTC_cnt"
  Relational Operator2/1 -> Terminator/1  "VDDM_MCUF1NoComDFS_flg"
  Constant12/1 -> Relational Operator2/2
  Logical Operator2/1 -> Logical Operator10/1, Timer1/1
  [VPMM_SysPwrSta_enum] -> Equal44/1
  Equal1/1 -> OR6/1
  [VDDM_MCUF1NoCom_flg] -> Logical Operator24/1
  Constant99/1 -> Equal1/2
  Equal44/1 -> Logical Operator2/1
  Constant100/1 -> Equal45/2
  [No_CAN3_BUS_OFF] -> Logical Operator2/2
  [VPMM_DrivetrainSelect_enum] -> Equal45/1
  OR6/1 -> Logical Operator2/4
  Equal45/1 -> OR6/2
  Constant1/1 -> Equal44/2
  [VPMM_DrivetrainSelect_enum] -> Equal1/1
  [VDDM_MCUF1NoCom_flg] -> Logical Operator30/3
  Equal21/1 -> Logical Operator30/1
  [No_CAN3_BUS_OFF] -> Logical Operator30/2
  Timer1/1 -> Equal28/1
  [VDDM_MCUF1NoComDet_flg] -> DTC_Couter1/1
  [VPMM_SysPwrSta_enum] -> Equal21/1
  Constant70/1 -> Timer1/4
  [task_time_s] -> Timer1/3
  Test Detection Criteria1/1 -> [VDDM_MCUF1NoComDet_flg]  "VDDM_MCUF1NoComDet_flg"
  Constant62/1 -> Equal21/2
  Constant69/1 -> Equal28/2
  Equal28/1 -> [VDDM_MCUF1NoComPass_flg]  "VDDM_MCUF1NoComPass_flg"
  [task_time_s] -> Test Detection Criteria1/2
  Constant68/1 -> Test Detection Criteria1/3
  Constant71/1 -> Test Detection Criteria1/4
  Constant14/1 -> DTC_Couter1/3
  [VDDM_MCUF1NoComCFSRls_flg] -> DTC_Couter1/2
  [VPMM_SysPwrSta_enum] -> Equal5/1
  Equal5/1 -> Logical Operator14/1
  Constant19/1 -> Test Detection Criteria2/4
  Timer2/1 -> Equal6/1
  Equal6/1 -> [VDDM_MCUR1NoComPass_flg]  "VDDM_MCUR1NoComPass_flg"
  Test Detection Criteria2/1 -> [VDDM_MCUR1NoComDet_flg]  "VDDM_MCUR1NoComDet_flg"
  Constant16/1 -> Test Detection Criteria2/3
  [VDDM_MCUR1NoCom_flg] -> Logical Operator14/3
  Constant18/1 -> Timer2/4
  Constant9/1 -> Equal5/2
  [No_CAN3_BUS_OFF] -> Logical Operator14/2
  [task_time_s] -> Test Detection Criteria2/2
  Constant17/1 -> Equal6/2
  [task_time_s] -> Timer2/3
  [VDDM_MCUF1NoComCFS_flg] -> DTC_Info/3
  [VDDM_MCUF1NoComPass_flg] -> DTC_Info/2
  [VDDM_MCUF1NoComDet_flg] -> DTC_Info/1
  DTC_Info/1 -> VDDM_MCUF1NoComDTC_raw32/1  "VDDM_MCUF1NoComDTC_raw32"
  [VDDM_MCUR1NoComDet_flg] -> DTC_Info1/1
  DTC_Info1/1 -> VDDM_MCUR1NoComDTC_raw32/1  "VDDM_MCUR1NoComDTC_raw32"
  [VDDM_MCUR1NoComCFS_flg] -> DTC_Info1/3
  [VDDM_MCUR1NoComPass_flg] -> DTC_Info1/2
  task_time_s/1 -> [task_time_s]
  VPMM_SysPwrSta_enum/1 -> [VPMM_SysPwrSta_enum]
  No_CAN3_BUS_OFF/1 -> [No_CAN3_BUS_OFF]
  VDDM_MCUF1NoCom_flg/1 -> [VDDM_MCUF1NoCom_flg]
  DTC_clear_request/1 -> [DTC_clear_request]
  VDDM_MCUR1NoCom_flg/1 -> [VDDM_MCUR1NoCom_flg]
  DTC_Couter1/1 -> [VDDM_MCUF1NoComCFS_flg]  "VDDM_MCUF1NoComCFS_flg"
  [DTC_clear_request] -> DTC_Info/4
  [DTC_clear_request] -> DTC_Info1/4
  [VDDM_MCUF1NoComCFSRls_flg] -> Switch6/2
  Switch6/1 -> Test Detection Criteria1/1
  Constant22/1 -> Switch6/1
  Logical Operator30/1 -> Switch6/3
  [VDDM_MCUR1NoComCFSRls_flg] -> Switch1/2
  Switch1/1 -> Test Detection Criteria2/1
  Constant23/1 -> Switch1/1
  [VPMM_SysPwrSta_enum] -> Equal11/1
  [No_CAN3_BUS_OFF] -> Logical Operator31/2
  Logical Operator37/1 -> Timer3/2
  [VPMM_SysPwrSta_enum] -> Equal16/1
  Timer3/1 -> Equal13/1
  Constant48/1 -> Equal13/2
  Logical Operator7/1 -> Timer4/1, Logical Operator26/1
  Test Detection Criteria3/1 -> [VDDM_MCUF1RCErrDet_flg]  "VDDM_MCUF1RCErrDet_flg"
  Constant51/1 -> Test Detection Criteria3/4
  Equal11/1 -> Logical Operator31/1
  Constant50/1 -> Timer3/4
  Constant34/1 -> Test Detection Criteria4/4
  Constant46/1 -> Equal11/2
  Equal17/1 -> [VDDM_MCUR1RCErrPass_flg]  "VDDM_MCUR1RCErrPass_flg"
  [VDDM_MCUF1RCErr_flg] -> Logical Operator31/3
  Test Detection Criteria4/1 -> [VDDM_MCUR1RCErrDet_flg]  "VDDM_MCUR1RCErrDet_flg"
  DTC_Info2/1 -> VDDM_MCUF1RCErrDTC_raw32/1  "VDDM_MCUF1RCErrDTC_raw32"
  [VDDM_MCUF1RCErrDet_flg] -> DTC_Info2/1
  [VDDM_MCUF1RCErrPass_flg] -> DTC_Info2/2
  DTC_Info3/1 -> VDDM_MCUR1RCErrDTC_raw32/1  "VDDM_MCUR1RCErrDTC_raw32"
  [task_time_s] -> Timer4/3
  [task_time_s] -> Test Detection Criteria3/2
  [VDDM_MCUR1RCErrPass_flg] -> DTC_Info3/2
  Timer4/1 -> Equal17/1
  [VDDM_MCUR1RCErrDet_flg] -> DTC_Info3/1
  [VDDM_MCUR1RCErr_flg] -> Logical Operator23/3
  Constant33/1 -> Timer4/4
  [VDDM_MCUF1RCErrCFSRls_flg] -> Switch3/2
  Constant53/1 -> Equal16/2
  Constant47/1 -> Test Detection Criteria3/3
  [task_time_s] -> Timer3/3
  Equal13/1 -> [VDDM_MCUF1RCErrPass_flg]  "VDDM_MCUF1RCErrPass_flg"
  Equal16/1 -> Logical Operator23/1
  [VDDM_MCUR1RCErrCFS_flg] -> DTC_Info3/3
  Logical Operator12/1 -> Timer3/1, Logical Operator37/1
  Constant32/1 -> Equal17/2
  [VDDM_MCUF1RCErrCFS_flg] -> DTC_Info2/3
  Constant38/1 -> Switch3/1
  [No_CAN3_BUS_OFF] -> Logical Operator23/2
  Switch3/1 -> Test Detection Criteria3/1
  Logical Operator26/1 -> Timer4/2
  Constant31/1 -> Test Detection Criteria4/3
  [VDDM_MCUR1RCErrCFSRls_flg] -> Switch2/2
  [task_time_s] -> Test Detection Criteria4/2
  Switch2/1 -> Test Detection Criteria4/1
  Constant39/1 -> Switch2/1
  [DTC_clear_request] -> DTC_Info2/4
  [DTC_clear_request] -> DTC_Info3/4
  [VPMM_SysPwrSta_enum] -> Equal24/1
  [No_CAN3_BUS_OFF] -> Logical Operator67/2
  Logical Operator70/1 -> Timer5/2
  [VPMM_SysPwrSta_enum] -> Equal29/1
  Timer5/1 -> Equal25/1
  Constant37/1 -> Equal25/2
  Logical Operator40/1 -> Logical Operator61/1, Timer6/1
  Test Detection Criteria5/1 -> [VDDM_MCUF1CSErrDet_flg]  "VDDM_MCUF1CSErrDet_flg"
  Constant84/1 -> Test Detection Criteria5/4
  Equal24/1 -> Logical Operator67/1
  Constant83/1 -> Timer5/4
  Constant65/1 -> Test Detection Criteria6/4
  Constant79/1 -> Equal24/2
  Equal30/1 -> [VDDM_MCUR1CSErrPass_flg]  "VDDM_MCUR1CSErrPass_flg"
  [VDDM_MCUF1CSErr_flg] -> Logical Operator67/3
  Test Detection Criteria6/1 -> [VDDM_MCUR1CSErrDet_flg]  "VDDM_MCUR1CSErrDet_flg"
  DTC_Info4/1 -> VDDM_MCUF1CSErrDTC_raw32/1  "VDDM_MCUF1CSErrDTC_raw32"
  [VDDM_MCUF1CSErrDet_flg] -> DTC_Info4/1
  [VDDM_MCUF1CSErrPass_flg] -> DTC_Info4/2
  DTC_Info5/1 -> VDDM_MCUR1CSErrDTC_raw32/1  "VDDM_MCUR1CSErrDTC_raw32"
  [task_time_s] -> Timer6/3
  [task_time_s] -> Test Detection Criteria5/2
  [VDDM_MCUR1CSErrPass_flg] -> DTC_Info5/2
  Timer6/1 -> Equal30/1
  [VDDM_MCUR1CSErrDet_flg] -> DTC_Info5/1
  [VDDM_MCUR1CSErr_flg] -> Logical Operator58/3
  Constant64/1 -> Timer6/4
  [VDDM_MCUF1CSErrCFSRls_flg] -> Switch5/2
  Constant86/1 -> Equal29/2
  Constant80/1 -> Test Detection Criteria5/3
  [task_time_s] -> Timer5/3
  Equal25/1 -> [VDDM_MCUF1CSErrPass_flg]  "VDDM_MCUF1CSErrPass_flg"
  Equal29/1 -> Logical Operator58/1
  [VDDM_MCUR1CSErrCFS_flg] -> DTC_Info5/3
  Logical Operator27/1 -> Logical Operator70/1, Timer5/1
  Constant63/1 -> Equal30/2
  [VDDM_MCUF1CSErrCFS_flg] -> DTC_Info4/3
  Constant73/1 -> Switch5/1
  [No_CAN3_BUS_OFF] -> Logical Operator58/2
  Switch5/1 -> Test Detection Criteria5/1
  Logical Operator61/1 -> Timer6/2
  Constant61/1 -> Test Detection Criteria6/3
  [VDDM_MCUR1CSErrCFSRls_flg] -> Switch4/2
  [task_time_s] -> Test Detection Criteria6/2
  Switch4/1 -> Test Detection Criteria6/1
  Constant74/1 -> Switch4/1
  [DTC_clear_request] -> DTC_Info4/4
  [DTC_clear_request] -> DTC_Info5/4
  [VDDM_MCUF1NoComCFS_flg] -> Logical Operator81/1
  Logical Operator81/1 -> Logical Operator31/4
  Logical Operator82/1 -> Logical Operator23/4
  [VDDM_MCUR1NoComCFS_flg] -> Logical Operator82/1
  Logical Operator83/1 -> Logical Operator67/4
  [VDDM_MCUF1NoComCFS_flg] -> Logical Operator83/1
  Logical Operator84/1 -> Logical Operator58/4
  [VDDM_MCUR1NoComCFS_flg] -> Logical Operator84/1
  VDDM_MCUF1RCErr_flg/1 -> [VDDM_MCUF1RCErr_flg]
  VDDM_MCUF1CSErr_flg/1 -> [VDDM_MCUF1CSErr_flg]
  VDDM_MCUR1RCErr_flg/1 -> [VDDM_MCUR1RCErr_flg]
  VDDM_MCUR1CSErr_flg/1 -> [VDDM_MCUR1CSErr_flg]
  Logical Operator31/1 -> Switch3/3
  Logical Operator67/1 -> Switch5/3
  Logical Operator14/1 -> Switch1/3
  Logical Operator23/1 -> Switch2/3
  Logical Operator58/1 -> Switch4/3
  [VDDM_MCUF1NoComCFS_flg] -> VDDM_MCUF1NoComCFS_flg/1
  [VDDM_MCUF1CSErrCFS_flg] -> VDDM_MCUF1CSErrCFS_flg/1
  [VDDM_MCUR1CSErrCFS_flg] -> VDDM_MCUR1CSErrCFS_flg/1
  [VDDM_MCUR1RCErrCFS_flg] -> VDDM_MCUR1RCErrCFS_flg/1
  [VDDM_MCUR1NoComCFS_flg] -> VDDM_MCUR1NoComCFS_flg/1
  [VDDM_MCUF1RCErrCFS_flg] -> VDDM_MCUF1RCErrCFS_flg/1
  VPMM_DrivetrainSelect_enum/1 -> [VPMM_DrivetrainSelect_enum]
  Equal/1 -> OR/1
  Equal33/1 -> OR/2
  Constant87/1 -> Equal/2
  [VPMM_DrivetrainSelect_enum] -> Equal33/1
  Constant88/1 -> Equal33/2
  OR/1 -> Logical Operator30/4
  [VPMM_DrivetrainSelect_enum] -> Equal35/1
  Constant89/1 -> Equal34/2
  Equal35/1 -> OR1/2
  [VPMM_DrivetrainSelect_enum] -> Equal34/1
  OR1/1 -> Logical Operator31/5
  Constant90/1 -> Equal35/2
  Equal34/1 -> OR1/1
  [VPMM_DrivetrainSelect_enum] -> Equal37/1
  Constant92/1 -> Equal37/2
  Constant91/1 -> Equal36/2
  [VPMM_DrivetrainSelect_enum] -> Equal36/1
  Equal36/1 -> OR2/1
  Equal37/1 -> OR2/2
  OR2/1 -> Logical Operator67/5
  [VPMM_DrivetrainSelect_enum] -> Equal39/1
  Constant93/1 -> Equal38/2
  Equal39/1 -> OR3/2
  [VPMM_DrivetrainSelect_enum] -> Equal38/1
  OR3/1 -> Logical Operator14/4
  Constant94/1 -> Equal39/2
  Equal38/1 -> OR3/1
  Equal40/1 -> OR4/1
  Constant96/1 -> Equal41/2
  [VPMM_DrivetrainSelect_enum] -> Equal40/1
  Equal41/1 -> OR4/2
  Constant95/1 -> Equal40/2
  [VPMM_DrivetrainSelect_enum] -> Equal41/1
  OR4/1 -> Logical Operator23/5
  Constant97/1 -> Equal42/2
  [VPMM_DrivetrainSelect_enum] -> Equal43/1
  [VPMM_DrivetrainSelect_enum] -> Equal42/1
  Constant98/1 -> Equal43/2
  Equal42/1 -> OR5/1
  Equal43/1 -> OR5/2
  OR5/1 -> Logical Operator58/5
  [VPMM_DrivetrainSelect_enum] -> Equal/1
  [VDDM_MCUF1NoComCFS_flg] -> Logical Operator/1
  [VDDM_MCUF1RCErrCFS_flg] -> Logical Operator/2
  [VDDM_MCUF1CSErrCFS_flg] -> Logical Operator/3
  Logical Operator/1 -> VDDM_MCUF1Err_flg/1  "VDDM_MCUF1Err_flg"
  [VDDM_MCUR1NoComCFS_flg] -> Logical Operator43/1
  [VDDM_MCUR1RCErrCFS_flg] -> Logical Operator43/2
  [VDDM_MCUR1CSErrCFS_flg] -> Logical Operator43/3
  Logical Operator43/1 -> VDDM_MCUR1Err_flg/1  "VDDM_MCUR1Err_flg"
